simulink model "CH11_3B"  (Simulink 10.1)
settings: Solver=ode45  StartTime=0.0  StopTime=0.5  RelTol=1e-3  EnableMultiTasking=on
undefined symbols (not defined in the file or in its folder): Fs, sided, Two
libraries: dspsnks4 x2
settings Model: Creator=my2  LastModifiedBy=IT
settings DataIOCC: LimitDataPoints=on  SignalLoggingSaveFormat=ModelDataLogs
settings DebuggingCC: SolverPrmCheckMsg=warning  FcnCallInpInsideContextMsg=warning

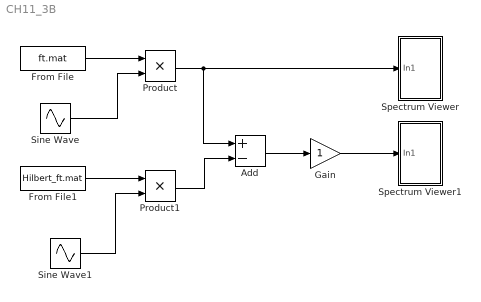
== system CH11_3B ==
  Add : Sum  Inputs=+-
  From File : FromFile  FileName=ft.mat  SampleTime=0
  From File1 : FromFile  FileName=Hilbert_ft.mat  SampleTime=0
  Gain : Gain
  Product : Product
  Product1 : Product
  Sine Wave : Sin  SampleTime=0
  Sine Wave1 : Sin  SampleTime=0
  Spectrum Viewer : Subsystem
  Spectrum Viewer1 : Subsystem
  wires:
  From File1/1 -> Product1/1
  From File/1 -> Product/1
  Sine Wave/1 -> Product/2
  Sine Wave1/1 -> Product1/2
  Product1/1 -> Add/2
  Product/1 -> Add/1, Spectrum Viewer/1(In1)
  Add/1 -> Gain/1
  Gain/1 -> Spectrum Viewer1/1(In1)

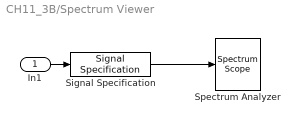
== system CH11_3B/Spectrum Viewer ==
  In1 : Inport
  Signal Specification : SignalSpecification  SampleTime=1/16e4
  Spectrum Analyzer : dspsnks4/Spectrum Scope  SystemSampleTime=-1  ScopeProperties=on  Domain=Frequency  HorizSpan=1  UseBuffer=on  BufferSize=1024  Overlap=64  inpFftLenInherit=on  FFTlength=1024  numAvg=200  DisplayProperties=off  AxisGrid=on  Memory=off  FrameNumber=on  AxisLegend=off  AxisZoom=off  OpenScopeAtSimStart=on  OpenScopeImmediately=off  FigPos="[549  354  800  160]"  AxisProperties=off  XUnits=Hertz  XRange=Two-sided ((-Fs/2...Fs/2])  XDisplay=0  InheritXIncr=on  XIncr=1.0  XLabel=Samples  XLimit=Auto  YUnits=dBm  XMax=1  XMin=0  YLabel=Magnitude-squared, dB  LineProperties=off  wintypeSpecScope=Hann  RsSpecScope=50  betaSpecScope=5  winsampSpecScope=Symmetric  XAxisParamsVer=6.9
      settings: SourceProductBaseCode=DS  YMin=-40  YMax=25
  wires:
  In1/1 -> Signal Specification/1
  Signal Specification/1 -> Spectrum Analyzer/1

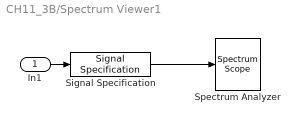
== system CH11_3B/Spectrum Viewer1 ==
  In1 : Inport
  Signal Specification : SignalSpecification  SampleTime=1/16e4
  Spectrum Analyzer : dspsnks4/Spectrum Scope  SystemSampleTime=-1  ScopeProperties=on  Domain=Frequency  HorizSpan=1  UseBuffer=on  BufferSize=1024  Overlap=64  inpFftLenInherit=on  FFTlength=1024  numAvg=200  DisplayProperties=off  AxisGrid=on  Memory=off  FrameNumber=on  AxisLegend=off  AxisZoom=off  OpenScopeAtSimStart=on  OpenScopeImmediately=off  FigPos="[549  354  800  160]"  AxisProperties=off  XUnits=Hertz  XRange=Two-sided ((-Fs/2...Fs/2])  XDisplay=0  InheritXIncr=on  XIncr=1.0  XLabel=Samples  XLimit=Auto  YUnits=dBm  XMax=1  XMin=0  YLabel=Magnitude-squared, dB  LineProperties=off  wintypeSpecScope=Hann  RsSpecScope=50  betaSpecScope=5  winsampSpecScope=Symmetric  XAxisParamsVer=6.9
      settings: SourceProductBaseCode=DS  YMin=-40  YMax=25
  wires:
  In1/1 -> Signal Specification/1
  Signal Specification/1 -> Spectrum Analyzer/1
